simulink model "untitled"  (R2022a)
settings: Solver=FixedStepAuto  StartTime=0.0  StopTime=2  FixedStep=1e-6  RelTol=1e-3
libraries: simulink x2, spsDCVoltageSourceLib x1, spsPermanentMagnetSynchronousMachineLib x1, spsTwoLevelConverterLib x1, spspowerguiLib x1
settings Model: Creator=Mengyang  LastModifiedBy=Mengyang

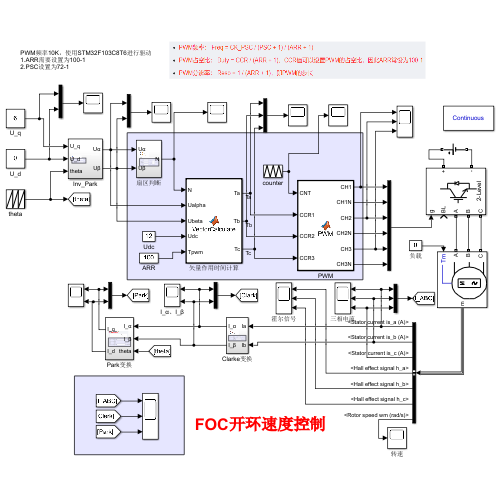
[thumbnail: Simulink's stored preview of the top-level diagram]
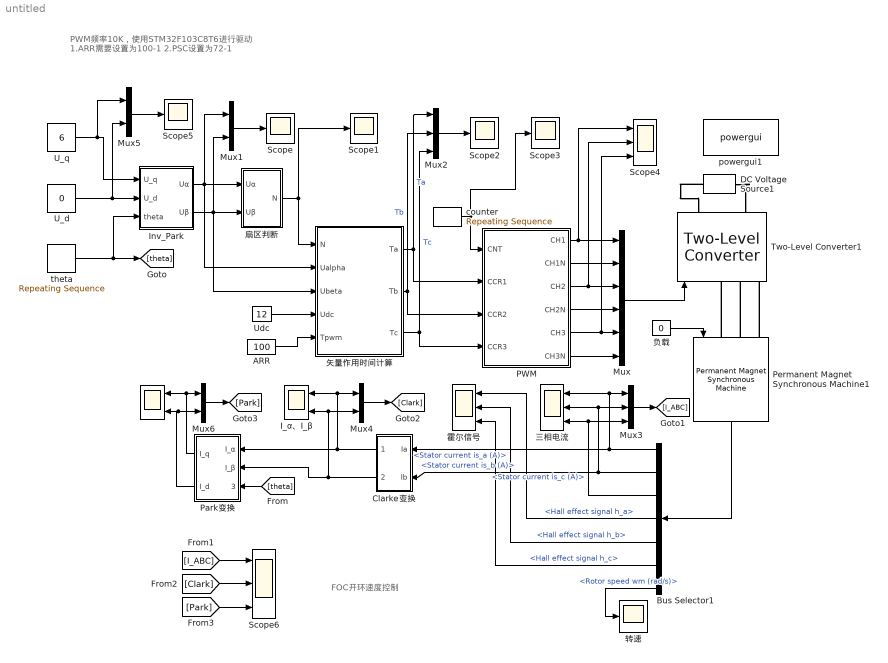
== system untitled ==
  note: PWM频率10K，使用STM32F103C8T6进行驱动
      | 1.ARR需要设置为100-1
      | 2.PSC设置为72-1
  note: FOC开环速度控制
  " " : Scope  NumInputPorts=2
  ARR : Constant  Value=100
  Bus Selector1 : BusSelector  OutputSignals=Stator current is_a (A),Stator current is_b (A),Stator current is_c (A),Hall effect signal h_a,Hall effect signal h_b,Hall effect signal h_c,Rotor speed wm (rad/s)
  Clarke变换 : Subsystem
  DC Voltage Source1 : spsDCVoltageSourceLib/DC Voltage Source  Amplitude=12  Measurements=None
  I_α、I_β : Scope  NumInputPorts=2
  Inv_Park : Subsystem
  Mux : Mux  Inputs=6
  Mux{1,4..6} (4 alike) : Mux  Inputs=2
  Mux2 : Mux  Inputs=3
  Mux3 : Mux  Inputs=3
  PWM : MATLAB Function  TreatAsAtomicUnit=on
  Park变换 : Subsystem
  Permanent Magnet Synchronous Machine1 : spsPermanentMagnetSynchronousMachineLib/Permanent Magnet Synchronous Machine  NbPhases=3  FluxDistribution=Sinusoidal  RotorType=Round  MechanicalLoad=Torque Tm  PresetModel=No  ShowDetailedParameters=on  MeasurementBus=off  Resistance=0.0485  Inductance=8.5e-3  dqInductances=[8.5e-3,8.5e-3]  La=0.000395  MachineConstant=Flux linkage established by magnets (V.s)  Flux=0.1194  VoltageCst=86.6271  TorqueCst=0.7164  Flat=120  Mechanical=[0.0027 0.0004924 4 0]  PolePairs=4  InitialConditions=[0,0, 0,0]  InitialConditions5ph=[0 0 0 0 0 0]  RefAngle=Aligned with phase A axis (original Park)  IterativeDiscreteModel=Trapezoidal non iterative  TsBlock=-1  TsPowergui=0
  Scope{,1..3,5} (5 alike) : Scope
  Scope4 : Scope  NumInputPorts=3
  Scope6 : Scope  NumInputPorts=3
  Two-Level Converter1 : spsTwoLevelConverterLib/Two-Level Converter  ModelType=Switching devices  Ron=1e-3  Rs=1e6  Cs=inf  Vforward=[0,0]  Ron_Diode=1e-3  Rs_Diode=1e6  Cs_Diode=inf  Vf_Diode=1e-3  Rs_CurrentSource=inf  Ron_ACsource=1e-3
      settings: SourceProductBaseCode=PS
  U_d : Constant  Value=0
  U_q : Constant  Value=6
  Udc : Constant  Value=12
  "counter " : simulink/Sources/Repeating Sequence  rep_seq_t=[0 0.0001 0.0002]  rep_seq_y=[0 100 0]
  powergui1 : spspowerguiLib/powergui  Priority=1  SimulationMode=Continuous  SampleTime=0.000001  frequency=60  Iterations=50  frequencyindice=0  Pbase=100e6  ErrMax=1e-4  UnitsV=kV  UnitsW=MW  buscounter=0  FunctionMessages=off  echomessages=off  EnableUseOfTLC=off  CurrentSourceSwitches=off  DisableSnubberDevices=off  DisableRonSwitches=off  DisableVfSwitches=off  DisplayEquations=off  AutomaticDiscreteSolvers=off  SolverType=Tustin/Backward Euler (TBE)  Interpol=off  ExternalGateDelay=off  methode=off  Ts=100  x0status=blocks  SPID=on  SwTol=0  HookPort=off  NonlinearTolerance=1e-4  nMaxIteration=100  ContinueOnMaxIteration=off  RestoreLinks=warning  ResistiveCurrentMeasurement=off  Frange=[0:2:500]  Ylog=off  Xlog=on  ShowGrid=off  save=off  variable=ZData  structure=0  ZoomFFT=off  StartTime=0.0  cycles=1  DisplayStyle=1  fundamental=60  FreqAxis=off  MaxFrequency=1000  frequencyindicesteady=1  RmsSteady=1  display=off
  "theta " : simulink/Sources/Repeating Sequence  rep_seq_t=[0 1]  rep_seq_y=[0 2*pi]
  三相电流 : Scope  NumInputPorts=3
  扇区判断 : Subsystem
  矢量作用时间计算 : MATLAB Function  TreatAsAtomicUnit=on
  负载 : Constant  Value=0
  转速 : Scope
  霍尔信号 : Scope  NumInputPorts=3
  wires:
  U_q/1 -> Mux5/1, Inv_Park/1(U_q)
  U_d/1 -> Inv_Park/2(U_d), Mux5/2
  "theta "/1 -> [theta], Inv_Park/3(theta)
  Inv_Park/1(Uα) -> 矢量作用时间计算/2(Ualpha), Mux1/1, 扇区判断/1(Uα)
  Inv_Park/2(Uβ) -> 矢量作用时间计算/3(Ubeta), Mux1/2, 扇区判断/2(Uβ)
  Mux1/1 -> Scope/1
  扇区判断/1(N) -> 矢量作用时间计算/1(N), Scope1/1
  Udc/1 -> 矢量作用时间计算/4(Udc)
  ARR/1 -> 矢量作用时间计算/5(Tpwm)
  Mux2/1 -> Scope2/1
  矢量作用时间计算/2(Tb) -> Mux2/2, PWM/3(CCR2)  "Tb"
  矢量作用时间计算/1(Ta) -> PWM/2(CCR1), Mux2/1  "Ta"
  Mux5/1 -> Scope5/1
  矢量作用时间计算/3(Tc) -> Mux2/3, PWM/4(CCR3)  "Tc"
  "counter "/1 -> Scope3/1, PWM/1(CNT)
  PWM/1(CH1) -> Scope4/1, Mux/1
  PWM/2(CH1N) -> Mux/2
  PWM/3(CH2) -> Scope4/2, Mux/3
  PWM/4(CH2N) -> Mux/4
  PWM/5(CH3) -> Scope4/3, Mux/5
  PWM/6(CH3N) -> Mux/6
  Mux/1 -> Two-Level Converter1/1
  负载/1 -> Permanent Magnet Synchronous Machine1/1
  Permanent Magnet Synchronous Machine1/1 -> Bus Selector1/1
  Bus Selector1/1 -> Mux3/1, 三相电流/1, Clarke变换/1(Ia)  "<Stator current is_a (A)>"
  Bus Selector1/2 -> Clarke变换/2(Ib), Mux3/2, 三相电流/2  "<Stator current is_b (A)>"
  Bus Selector1/3 -> Mux3/3, 三相电流/3  "<Stator current is_c (A)>"
  Bus Selector1/4 -> 霍尔信号/1  "<Hall effect signal h_a>"
  Bus Selector1/5 -> 霍尔信号/2  "<Hall effect signal h_b>"
  Bus Selector1/6 -> 霍尔信号/3  "<Hall effect signal h_c>"
  Bus Selector1/7 -> 转速/1  "<Rotor speed wm (rad/s)>"
  Clarke变换/2(I_β) -> Mux4/2, I_α、I_β/2, Park变换/2(I_β)
  [theta] -> Park变换/3(theta)
  Park变换/1(I_q) -> Mux6/1, " "/1
  Park变换/2(I_d) -> Mux6/2, " "/2
  Mux3/1 -> [I_ABC]
  Clarke变换/1(I_α) -> Park变换/1(I_α), Mux4/1, I_α、I_β/1
  Mux4/1 -> [Clark]
  Mux6/1 -> [Park]
  [I_ABC] -> Scope6/1
  [Clark] -> Scope6/2
  [Park] -> Scope6/3
  connections:
  DC Voltage Source1/RConn1 -- Two-Level Converter1/RConn1
  DC Voltage Source1/LConn1 -- Two-Level Converter1/RConn2
  Permanent Magnet Synchronous Machine1/LConn1 -- Two-Level Converter1/LConn1
  Permanent Magnet Synchronous Machine1/LConn2 -- Two-Level Converter1/LConn2
  Permanent Magnet Synchronous Machine1/LConn3 -- Two-Level Converter1/LConn3

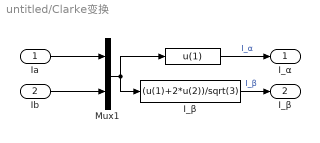
== system untitled/Clarke变换 ==
  Ia : Inport
  Ib : Inport  Port=2
  " " : Fcn  Expr=u(1)
  " I_β" : Fcn  Expr=(u(1)+2*u(2))/sqrt(3)
  Mux1 : Mux  Inputs=2
  I_α : Outport
  I_β : Outport  Port=2
  wires:
  Ia/1 -> Mux1/1
  Ib/1 -> Mux1/2
  " I_β"/1 -> I_β/1  "I_β"
  Mux1/1 -> " I_β"/1, " "/1
  " "/1 -> I_α/1  "I_α"

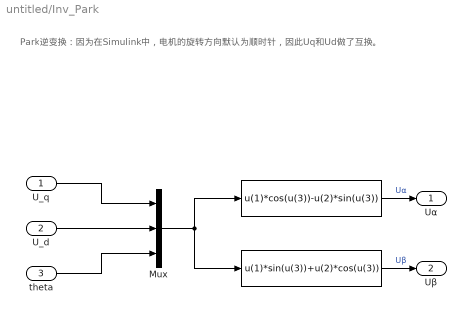
== system untitled/Inv_Park ==
  note: Park逆变换：因为在Simulink中，电机的旋转方向默认为顺时针，因此Uq和Ud做了互换。
  U_q : Inport
  U_d : Inport  Port=2
  theta : Inport  Port=3
  " " : Fcn  Expr=u(1)*cos(u(3))-u(2)*sin(u(3))
  "  " : Fcn  Expr=u(1)*sin(u(3))+u(2)*cos(u(3))
  Mux : Mux  Inputs=3
  Uα : Outport
  Uβ : Outport  Port=2
  wires:
  Mux/1 -> "  "/1, " "/1
  theta/1 -> Mux/3
  U_d/1 -> Mux/2
  "  "/1 -> Uβ/1  "Uβ"
  " "/1 -> Uα/1  "Uα"
  U_q/1 -> Mux/1

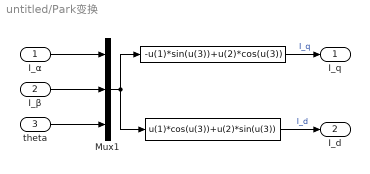
== system untitled/Park变换 ==
  I_α : Inport
  I_β : Inport  Port=2
  theta : Inport  Port=3
  " " : Fcn  Expr=-u(1)*sin(u(3))+u(2)*cos(u(3))
  "  " : Fcn  Expr=u(1)*cos(u(3))+u(2)*sin(u(3))
  Mux1 : Mux  Inputs=3
  I_q : Outport
  I_d : Outport  Port=2
  wires:
  I_α/1 -> Mux1/1
  I_β/1 -> Mux1/2
  "  "/1 -> I_d/1  "I_d"
  Mux1/1 -> " "/1, "  "/1
  " "/1 -> I_q/1  "I_q"
  theta/1 -> Mux1/3

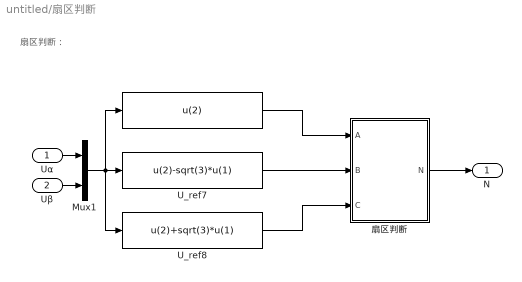
== system untitled/扇区判断 ==
  note: 扇区判断：
  Uα : Inport
  Uβ : Inport  Port=2
  " " : Fcn  Expr=u(2)
  Mux1 : Mux  Inputs=2
  U_ref7 : Fcn  Expr=u(2)-sqrt(3)*u(1)
  U_ref8 : Fcn  Expr=u(2)+sqrt(3)*u(1)
  扇区判断 : MATLAB Function  TreatAsAtomicUnit=on
  N : Outport
  wires:
  Mux1/1 -> U_ref8/1, U_ref7/1, " "/1
  Uα/1 -> Mux1/1
  Uβ/1 -> Mux1/2
  U_ref7/1 -> 扇区判断/2(B)
  " "/1 -> 扇区判断/1(A)
  U_ref8/1 -> 扇区判断/3(C)
  扇区判断/1(N) -> N/1

== matlab function untitled/矢量作用时间计算 ==
  data: N input; Ta output; Ualpha input; Ubeta input; Udc input; Tpwm input; Tb output; Tc output
function [Ta,Tb,Tc] = VectorCalculate(N,Ualpha,Ubeta,Udc,Tpwm)

Ta=double(0);
Tb=double(0);
Tc=double(0);

X=(sqrt(3)*Tpwm)/Udc*Ubeta;  % 系数1
Y=(sqrt(3)*Tpwm)/Udc*((sqrt(3)/2)*Ualpha+0.5*Ubeta); % 系数2
Z=(sqrt(3)*Tpwm)/Udc*(-(sqrt(3)/2)*Ualpha+0.5*Ubeta); % 系数3

M = (sqrt(3)/Udc)*Tpwm;
U1 = Ubeta*M;
U2 = ((sqrt(3)/2)*Ualpha-0.5*Ubeta)*M;
U3 = ((sqrt(3)/2)*Ualpha+0.5*Ubeta)*M;

%% 扇区1
if(N==5)  
   T4 = U2;
   T6 = U1;
   SUM = T4+T6;
   if(SUM>Tpwm)
       K_SVPWM = Tpwm/SUM;
       T4= K_SVPWM*T4;
       T6= K_SVPWM*T6;
   end
   T7=(Tpwm-T4-T6)/2;
   Ta = T4+T6+T7;
   Tb = T6+T7;
   Tc = T7;
end
%% 扇区2
if(N==7)  
   T2 = -U2;
   T6 = U3;
   SUM = T2+T6;
   if(SUM>Tpwm)
       K_SVPWM = Tpwm/SUM;
       T2= K_SVPWM*T2;
       T6= K_SVPWM*T6;
   end
   T7=(Tpwm-T2-T6)/2;
   Ta = T6+T7;
   Tb = T2+T6+T7;
   Tc = T7;
end
%% 扇区3
if(N==6)  
   T2 = U1;
   T3 = -U3;
   SUM = T2+T3;
   if(SUM>Tpwm)
       K_SVPWM = Tpwm/SUM;
       T2= K_SVPWM*T2;
       T3= K_SVPWM*T3;
   end
   T7=(Tpwm-T2-T3)/2;
   Ta = T7;
   Tb = T2+T3+T7;
   Tc = T3+T7;
end
%% 扇区4
if(N==2)  
   T1 = -U1;
   T3 = -U2;
   SUM = T1+T3;
   if(SUM>Tpwm)
       K_SVPWM = Tpwm/SUM;
       T1= K_SVPWM*T1;
       T3= K_SVPWM*T3;
   end
   T7=(Tpwm-T1-T3)/2;
   Ta = T7;
   Tb = T3+T7;
   Tc = T1+T3+T7;
end
%% 扇区5
if(N==0)  
   T1 = -U3;
   T5 = U2;
   SUM = T1+T5;
   if(SUM>Tpwm)
       K_SVPWM = Tpwm/SUM;
       T1= K_SVPWM*T1;
       T5= K_SVPWM*T5;
   end
   T7=(Tpwm-T1-T5)/2;
   Ta = T5+T7;
   Tb = T7;
   Tc = T1+T5+T7;
end
%% 扇区6
if(N==1)  
   T4 = U3;
   T5 = -U1;
   SUM = T4+T5;
   if(SUM>Tpwm)
       K_SVPWM = Tpwm/SUM;
       T4= K_SVPWM*T4;
       T5= K_SVPWM*T5;
   end
   T7=(Tpwm-T4-T5)/2;
   Ta = T4+T5+T7;
   Tb = T7;
   Tc = T5+T7;
end

== matlab function untitled/扇区判断/扇区判断 ==
  data: A input; N output; B input; C input
function N = SectorJudge(A,B,C)
N=0;

% N = 4A+2B+C
if(A>0)
    N=N+4;
end

if(B>0)
    N=N+2;
end

if(C>0)
    N=N+1;
end

== matlab function untitled/PWM ==
  data: CNT input; CH1 output; CCR1 input; CCR2 input; CCR3 input; CH1N output; CH2 output; CH2N output; CH3 output; CH3N output
function [CH1,CH1N,CH2,CH2N,CH3,CH3N] = PWM(CNT,CCR1,CCR2,CCR3)

if(CNT <= CCR1)
    CH1=0;
    CH1N=1;
else
    CH1=1;
    CH1N=0;
end

if(CNT <= CCR2)
    CH2=0;
    CH2N=1;
else
    CH2=1;
    CH2N=0;
end

if(CNT <= CCR3)
    CH3=0;
    CH3N=1;
else
    CH3=1;
    CH3N=0;
end
